simulink model "obs_primario_2015"  (R2015a)
settings: Solver=ode45  SolverMode=SingleTasking  StartTime=0.0  StopTime=10.0  RelTol=1e-3
undefined symbols (not defined in the file or in its folder): C, gama, Lk, phi
settings Model: CovMetricSettings=dwe  CovHtmlReporting=off  covSaveCumulativeToWorkspaceVar=off  CovSaveSingleToWorkspaceVar=off  CovExternalEMLEnable=on  Creator=Tiago  LastModifiedBy=Tiago
settings DataIOCC: LimitDataPoints=off  SaveFormat=Dataset  ReturnWorkspaceOutputs=on
settings DebuggingCC: SFUnexpectedBacktrackingDiag=error  SFNoUnconditionalDefaultTransitionDiag=error
settings HardwareCC: ProdBitPerPointer=64  ProdLargestAtomicFloat=Float  ProdIntDivRoundTo=Zero  ProdEndianess=LittleEndian  ProdHWDeviceType=Specified
settings ModelReferenceCC: PropagateSignalLabelsOutOfModel=on
settings SFSimCC: SimUseLocalCustomCode=on
settings RTWCC: RTWUseLocalCustomCode=on
settings GRTTargetCC: TargetLangStandard=C99 (ISO)  GeneratePreprocessorConditionals=Use local settings

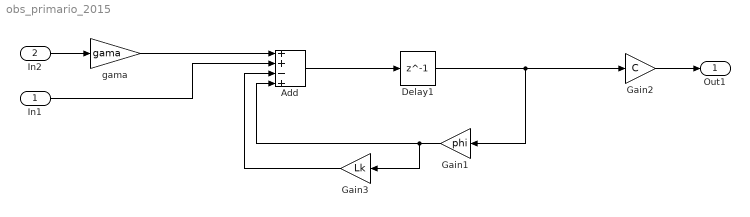
== system obs_primario_2015 ==
  In1 : Inport
  In2 : Inport  Port=2
  Add : Sum  Inputs=++-+
  Delay1 : Delay  DelayLength=1
  Gain1 : Gain  Gain=phi
  Gain2 : Gain  Gain=C
  Gain3 : Gain  Gain=Lk
  "gama " : Gain  Gain=gama
  Out1 : Outport
  wires:
  "gama "/1 -> Add/1
  Delay1/1 -> Gain2/1, Gain1/1
  Gain1/1 -> Add/4, Gain3/1
  In2/1 -> "gama "/1
  Add/1 -> Delay1/1
  Gain3/1 -> Add/3
  In1/1 -> Add/2
  Gain2/1 -> Out1/1
